simulink model "demoParkInvSILBlockRef"  (Simulink 8.1)
settings: Solver=FixedStepDiscrete  StartTime=0.0  StopTime=1000  FixedStep=.1  RelTol=1e-3
libraries: BAMLIB564xL x4, simulink_extras x3
settings Model: Creator=evarshavskaya  LastModifiedBy=evarshavskaya
settings DataIOCC: ExternalInput=off  InitialState=off  LimitDataPoints=off  SaveOutput=off  SignalLogging=off  SaveTime=off
settings OptimizationCC: InlineParams=on  OptimizeModelRefInitCode=on  LifeSpan=1
settings DebuggingCC: InheritedTsInSrcMsg=none  SingleTaskRateTransMsg=error  ParameterDowncastMsg=none  ParameterOverflowMsg=warning  ParameterPrecisionLossMsg=none  ParameterTunabilityLossMsg=none  InvalidFcnCallConnMsg=none  UnconnectedInputMsg=none  UnconnectedOutputMsg=none  UnconnectedLineMsg=none  BusObjectLabelMismatch=none  RootOutportRequireBusObject=none  UnknownTsInhSupMsg=error  ModelReferenceDataLoggingMessage=none  ModelReferenceExtraNoncontSigs=none  StrictBusMsg=None
settings HardwareCC: ProdIntDivRoundTo=Zero  ProdEndianess=BigEndian  ProdHWDeviceType=Generic->Custom  TargetIntDivRoundTo=Zero  TargetEndianess=BigEndian  TargetHWDeviceType=Generic->Custom
settings RTWCC: SystemTargetFile=ert.tlc  TemplateMakefile=ert_default_tmf  PostCodeGenCommand=rappid_analyzegencode(buildInfo)  Description=Embedded Coder  ProcessScript=ert_make_rtw_hook  PortableWordSizes=on
settings CodeAppCC: IgnoreCustomStorageClasses=off  MaxIdLength=63  CustomSymbolStrType=$N$R$M  InternalIdentifier=Classic
settings ERTTargetCC: CodeReplacementLibrary=ANSI_C  MultiwordLength=2048  GenerateSampleERTMain=on  SuppressErrorStatus=on  SupportAbsoluteTime=off  InlinedParameterPlacement=NonHierarchical  ERTCustomFileTemplate=example_file_process.tlc  ConvertIfToSwitch=off  SuppressUnreachableDefaultCases=off

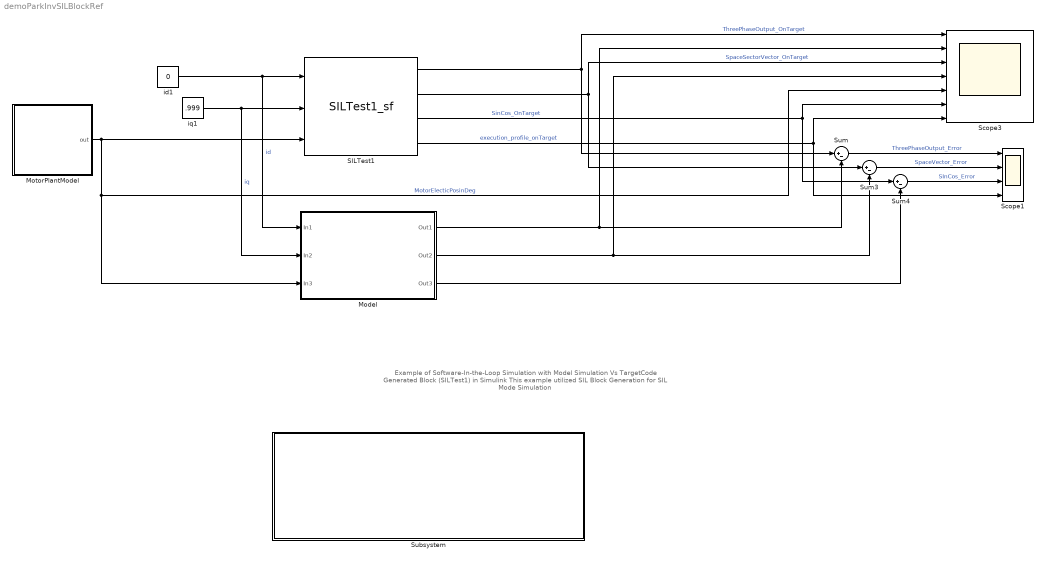
== system demoParkInvSILBlockRef ==
  note: Example of Software-In-the-Loop Simulation with Model Simulation Vs TargetCode Generated Block (SILTest1) in Simulink
      | This example utilized SIL Block Generation for SIL Mode Simulation
  Model : Subsystem
  MotorPlantModel : Stateflow chart  TreatAsAtomicUnit=on
  SILTest1 : S-Function  FunctionName=SILTest1_sf  SFunctionModules=""  EnableBusSupport=off  mask{rtw_sf_name=SILTest1_sf, showVar=off}
      mask prompts: rtw_sf_name "Generated S-function name (model_sf):"; showVar "Show module list"
      mask help: Simulink Coder generated S-function.
      mask init:
      | displist = '';
      | if ~strcmp(get_param(gcb, 'FunctionName'), rtw_sf_name);
      |   set_param(gcb, 'FunctionName', rtw_sf_name);
      | end
      | % Check if we are generating code
      | rtw_mode = false;
      | if strcmpi(get_param(bdroot(gcb),'SimulationStatus'),'Initializing')
      | 	rtw_mode = strcmpi(get_param(bdroot(gcb),'BuildingRTWCode'),'on') && ...
      | 		~strcmpi(get_param(bdroot(gcb),'TargetStyle'),'SimulationTarget');
      | end
      | if showVar || rtw_mode
      | 	if exist('rtwsfunc') == 2 | exist('rtwsfunc') == 6
      | 		tmplist = rtwsfunc(rtw_sf_name,gcb);
      | 		tmplist = ['\nList of Modules:\n', tmplist];
      | 	elseif showVar
      | 		tmplist = '\nList of Modules:\nNot licensed\n';
      |  	end
      | end
      | if showVar
      |   displist = tmplist;
      | end
      settings: CopyFcn=|
      | if ~strcmp(get_param(gcb,'Linkstatus'),'none') && ...
      | ~strcmp(get_param(gcb,'Linkstatus'),'implicit')
      |   set_param(gcb,'LinkStatus','none');
      | end
      mask Help: helpview([docroot '/toolbox/ecoder/helptargets.map'], 'SIL_block');
      mask Display:
      | port_label('input',1,'In1');
      | port_label('input',2,'In2');
      | port_label('input',3,'In3');
      | port_label('output',1,'Out1');
      | port_label('output',2,'Out2');
      | port_label('output',3,'Out3');
      | port_label('output',4,'Out4');
  Scope1 : Scope  NumInputPorts=4
      settings: TimeRange=20  YMin=5.55112e-017~5.55112e-017~1~1  YMax=1~1~6~6
  Scope3 : Scope  NumInputPorts=7
      settings: TimeRange=20  YMin=5.55112e-017~5.55112e-017~1~1~0~-1~220  YMax=1~1~6~6~400~1~320  SaveName=ScopeData2
  Subsystem : Subsystem
      settings: OpenFcn=|
      | open_system('SILTest1.mdl');
      | rappid_564xl_set_pilsil_mode('SILTest1','silblock');
      mask Display:
      | crlf =sprintf('\n');
      | st=['1. Click on this block to generate SIL Block, Run model!'];
      | disp(st);
  Sum : Sum  Inputs=|+-
  Sum3 : Sum  Inputs=|+-
  Sum4 : Sum  Inputs=|+-
  id1 : Constant  Value=0  OutDataTypeStr=single
  iq1 : Constant  Value=.999  OutDataTypeStr=single
  wires:
  SILTest1/1 -> Scope3/1, Sum/1  "ThreePhaseOutput_OnTarget"
  SILTest1/2 -> Scope3/3, Sum3/1  "SpaceSectorVector_OnTarget"
  SILTest1/3 -> Scope3/6, Sum4/1  "SinCos_OnTarget"
  MotorPlantModel/1(out) -> Scope3/5, Model/3(In3), SILTest1/3  "MotorElecticPosinDeg"
  id1/1 -> SILTest1/1, Model/1(In1)  "id"
  iq1/1 -> Model/2(In2), SILTest1/2  "iq"
  Model/1(Out1) -> Scope3/2, Sum/2
  Model/2(Out2) -> Scope3/4, Sum3/2
  SILTest1/4 -> Scope3/7, Scope1/4  "execution_profile_onTarget"
  Sum/1 -> Scope1/1  "ThreePhaseOutput_Error"
  Sum3/1 -> Scope1/2  "SpaceVector_Error"
  Model/3(Out3) -> Sum4/2
  Sum4/1 -> Scope1/3  "SInCos_Error"

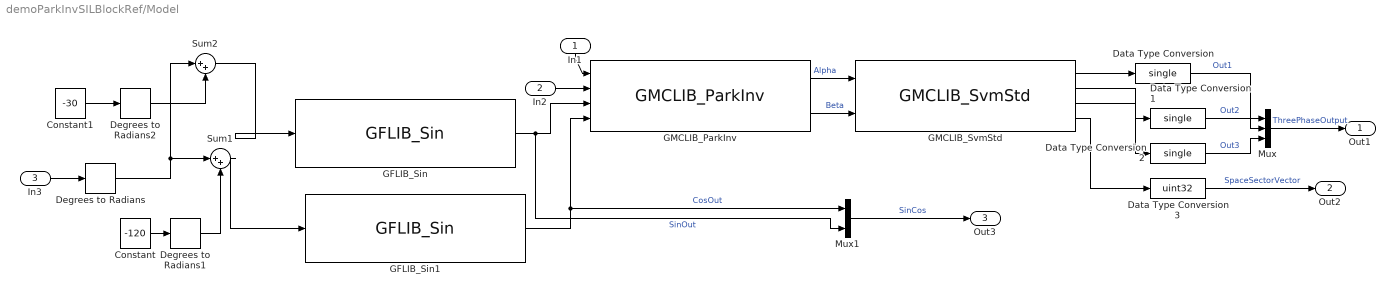
== system demoParkInvSILBlockRef/Model ==
  In1 : Inport
  In2 : Inport  Port=2
  In3 : Inport  Port=3
  Constant : Constant  Value=-120  OutDataTypeStr=single
  Constant1 : Constant  Value=-30  OutDataTypeStr=single
  Data Type Conversion : DataTypeConversion  OutDataTypeStr=single
  Data Type Conversion1 : DataTypeConversion  OutDataTypeStr=single
  Data Type Conversion2 : DataTypeConversion  OutDataTypeStr=single
  Data Type Conversion3 : DataTypeConversion  OutDataTypeStr=uint32
  Degrees to Radians : simulink_extras/Transformations/Degrees to Radians  SystemSampleTime=-1
  Degrees to Radians1 : simulink_extras/Transformations/Degrees to Radians  SystemSampleTime=-1
  Degrees to Radians2 : simulink_extras/Transformations/Degrees to Radians  SystemSampleTime=-1
  GFLIB_Sin : BAMLIB564xL/General Functions/GFLIB_Sin  SystemSampleTime=-1
  GFLIB_Sin1 : BAMLIB564xL/General Functions/GFLIB_Sin  SystemSampleTime=-1
  GMCLIB_ParkInv : BAMLIB564xL/General Motor Control Functions/GMCLIB_ParkInv  SystemSampleTime=-1
  GMCLIB_SvmStd : BAMLIB564xL/General Motor Control Functions/GMCLIB_SvmStd  SystemSampleTime=-1
  Mux : Mux  Inputs=3
  Mux1 : Mux  Inputs=2
  Sum1 : Sum  Inputs=|++
  Sum2 : Sum  Inputs=|++
  Out1 : Outport
  Out2 : Outport  Port=2
  Out3 : Outport  Port=3
  wires:
  Data Type Conversion/1 -> Mux/1  "Out1"
  Data Type Conversion1/1 -> Mux/2  "Out2"
  Data Type Conversion2/1 -> Mux/3  "Out3"
  GFLIB_Sin/1 -> GMCLIB_ParkInv/3, Mux1/2  "SinOut"
  GFLIB_Sin1/1 -> GMCLIB_ParkInv/4, Mux1/1  "CosOut"
  GMCLIB_SvmStd/4 -> Data Type Conversion3/1
  GMCLIB_SvmStd/3 -> Data Type Conversion2/1
  GMCLIB_SvmStd/2 -> Data Type Conversion1/1
  GMCLIB_SvmStd/1 -> Data Type Conversion/1
  GMCLIB_ParkInv/2 -> GMCLIB_SvmStd/2  "Beta"
  GMCLIB_ParkInv/1 -> GMCLIB_SvmStd/1  "Alpha"
  Sum2/1 -> GFLIB_Sin/1
  Sum1/1 -> GFLIB_Sin1/1
  Degrees to Radians2/1 -> Sum2/2
  Constant1/1 -> Degrees to Radians2/1
  Degrees to Radians1/1 -> Sum1/2
  Constant/1 -> Degrees to Radians1/1
  Degrees to Radians/1 -> Sum2/1, Sum1/1
  In1/1 -> GMCLIB_ParkInv/1
  In2/1 -> GMCLIB_ParkInv/2
  In3/1 -> Degrees to Radians/1
  Mux/1 -> Out1/1  "ThreePhaseOutput"
  Data Type Conversion3/1 -> Out2/1  "SpaceSectorVector"
  Mux1/1 -> Out3/1  "SinCos"

== system demoParkInvSILBlockRef/Subsystem ==

== stateflow chart MotorPlantModel ==
  settings: sampleTime=1/360
  state Normal
    en:out=1;
    du:out=out+1;
  Normal -> Normal : [out >= 360]
  (default) -> Normal
  data: out output single
